simulink model "protorype_multiple_msg"  (R2021b)
settings: Solver=FixedStepAuto  StartTime=0.0  StopTime=151  FixedStep=50  RelTol=1e-3
settings Model: Creator=vgaggero  LastModifiedBy=vgaggero

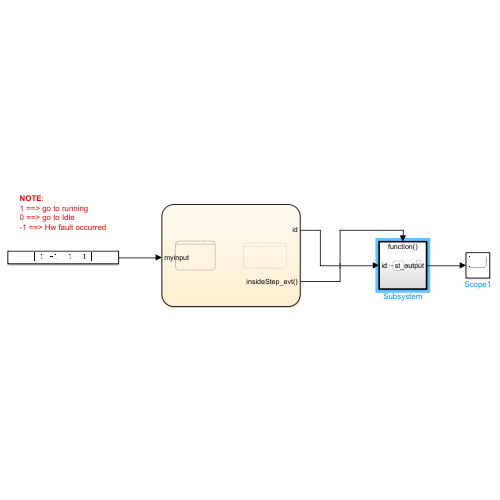
[thumbnail: Simulink's stored preview of the top-level diagram]
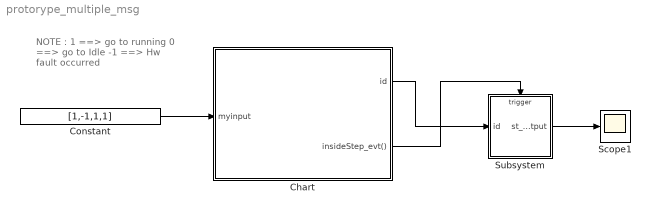
== system protorype_multiple_msg ==
  note: NOTE :
      | 1 ==> go to running
      | 0 ==> go to Idle
      | -1 ==> Hw fault occurred
  Chart : Stateflow chart  TreatAsAtomicUnit=on
  Constant : Constant  Value=[1,-1,1,1]  OutDataTypeStr=int32
  Scope1 : Scope
  Subsystem : Subsystem
  wires:
  Constant/1 -> Chart/1(myinput)
  Chart/2(insideStep_evt()) -> Subsystem/Trigger
  Chart/1(id) -> Subsystem/1(id)
  Subsystem/1(st_output) -> Scope1/1

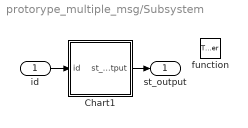
== system protorype_multiple_msg/Subsystem ==
  id : Inport
  function : TriggerPort  TriggerType=function-call  VariantControl=(inherit)
  Chart1 : Stateflow chart  TreatAsAtomicUnit=on
  st_output : Outport
  wires:
  Chart1/1(st_output) -> st_output/1
  id/1 -> Chart1/1(id)

== stateflow chart protorype_multiple_msg/Subsystem/Chart1 ==
  state Idle
    entry:
    st_output=0;
  state Running
    entry:
    st_output=100;
  state HwFault
    entry:
    st_output=-100;
  (default) -> Idle
  Idle -> Running : [id==1]
  HwFault -> Idle : [id==0]
  Running -> HwFault : [id==-1]
  data: st_output output int32 size=1; id input int32 size=1

== stateflow chart protorype_multiple_msg/Chart ==
  state for_loop [parallel]
    settings: executionOrder=1
    state init
      entry:
      id=0;
    (default) -> init
    (junction 19) -> init
    init -> (junction 7) : {index=1}
    (junction 7) -> (junction 9) [order 1] : [index<5]
    (junction 9) -> (junction 11) : {id=myinput(index);send(insideStep_evt);}
    (junction 11) -> (junction 7) : {index = index + 1}
    (junction 7) -> (junction 19) [order 2]
  state my_state_machine [parallel] [commented out]
    state Home [commented out]
      entry:
      output=100;
      du:
      output=index;
    (default) -> Home [commented out]
    Home -> Home [commented out] : [insideStep_evt]{output=output+1;}
  data: myinput input int32 size=4; index local int32 size=1; id output int32 size=1 =int32(0); data local int32 =int32(0)
  events: insideStep_evt output FUNCTION_CALL_EVENT
